simulink model "pole_placement_ctrl"  (R2025b)
settings: Solver=VariableStepAuto  StartTime=0.0  StopTime=100  RelTol=1e-3
values from neighbouring files (symbols this model uses):
  A = [0 1 0 0;     (m_b*g*r^2)/(I_b*l) 0 (m_b*g*r^2)/(I_b) 0 ;      0 0 0 1;    20 0 (M_r*d*g)/I_r 0 ]    [Copy_of_LQR_ctrl.m]    (also in LQR_ctrl.m = [0 1 0 0;     A1(1,1) 0 A1(1,2) 0;     0 0 0 1;    A1(2,1) 0; Rlocus_ctrl.m = [0 1 0 0;     A1(1,1) 0 A1(1,2) 0;     0 0 0 1;     A1(2,1) ; State4.m = [0 1 0 0;     A1(1,1) 0 A1(1,2) 0;     0 0 0 1;     A1(2,1) ; pole_placement_ctrl.m = [0 1 0 0;     A1(1,1) 0 A1(1,2) 0;     0 0 0 1;     A1(2,1) )
  B = -[0 ; 0; 0 ; ((I_w/R) + (M_w+M_r)*R)/(I_r)]    [Copy_of_LQR_ctrl.m]    (also in LQR_ctrl.m = -[0 ; B1(1); 0 ; B1(2)]; Rlocus_ctrl.m = -[0 ; B1(1); 0 ; B1(2)]; State4.m = -[0 ; B1(1); 0 ; B1(2)]; pole_placement_ctrl.m = -[0 ; B1(1); 0 ; B1(2)])
  C = [0 0 1 0]    [Copy_of_LQR_ctrl.m]    (also in LQR_ctrl.m; Rlocus_ctrl.m = Kpi * C_pi; State4.m = eye(4); pole_placement_ctrl.m = eye(4))
  D = [0]    [Copy_of_LQR_ctrl.m]    (also in LQR_ctrl.m; Rlocus_ctrl.m = zeros(4,1); State4.m = zeros(4,1); pole_placement_ctrl.m = zeros(4,1))
  K = lqr(A, B, Q, R)    [LQR_ctrl.m]    (also in Rlocus_ctrl.m = place(A,B,poles); State4.m; pole_placement_ctrl.m = place(A,B,poles))
settings Model: Creator=Abhi  LastModifiedBy=Abhi

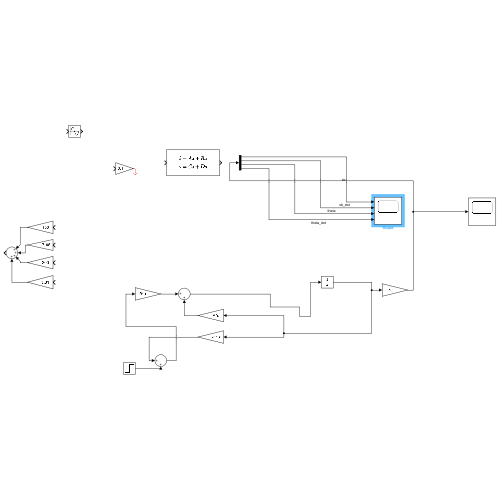
[thumbnail: Simulink's stored preview of the top-level diagram]
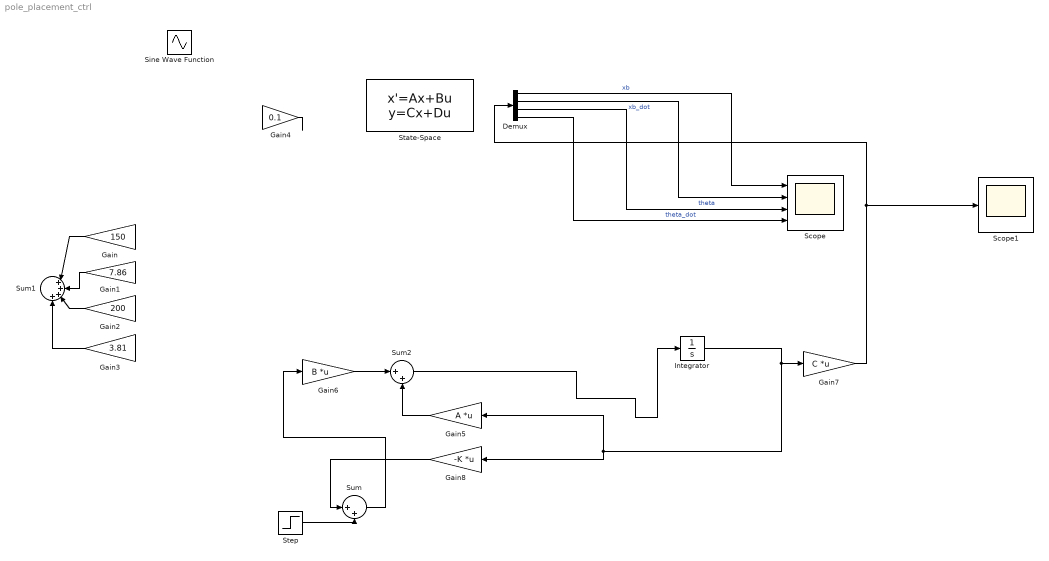
== system pole_placement_ctrl ==
  Demux : Demux
  Gain : Gain  Gain=150
  Gain1 : Gain  Gain=7.86
  Gain2 : Gain  Gain=200
  Gain3 : Gain  Gain=3.81
  Gain4 : Gain  Gain=0.1
  Gain5 : Gain  Gain=A  Multiplication=Matrix(K*u)
  Gain6 : Gain  Gain=B  Multiplication=Matrix(K*u)
  Gain7 : Gain  Gain=C  Multiplication=Matrix(K*u)
  Gain8 : Gain  Gain=-K  Multiplication=Matrix(K*u)
  Integrator : Integrator  InitialCondition=[0;0;0;0]
  Scope : Scope  NumInputPorts=4
      settings: ActiveDisplayYMinimum=-0.000176557833233224  ActiveDisplayYMaximum=0.0014372539888235084
  Scope1 : Scope
      settings: ActiveDisplayYMinimum=-0.034416313803153124  ActiveDisplayYMaximum=0.077437500890314079
  Sine Wave Function : Sin  TimeSource=Use external signal  SampleTime=0
  State-Space : StateSpace  A=A-B*K  B=zeros(4)  C=C-D*K  D=zeros(4)  InitialCondition=[0;0;0;0]
  Step : Step  SampleTime=0
  Sum : Sum  Inputs=|++
  Sum1 : Sum  Inputs=|++++
  Sum2 : Sum  Inputs=|++
  wires:
  Demux/3 -> Scope/3  "theta"
  Demux/1 -> Scope/1  "xb"
  Demux/4 -> Scope/4  "theta_dot"
  Demux/2 -> Scope/2  "xb_dot"
  Gain/1 -> Sum1/1
  Gain1/1 -> Sum1/2
  Gain2/1 -> Sum1/3
  Gain3/1 -> Sum1/4
  Gain4/1 -> ?
  Sum2/1 -> Integrator/1
  Integrator/1 -> Gain5/1, Gain8/1, Gain7/1
  Gain7/1 -> Scope1/1, Demux/1
  Gain6/1 -> Sum2/1
  Gain5/1 -> Sum2/2
  Step/1 -> Sum/2
  Gain8/1 -> Sum/1
  Sum/1 -> Gain6/1
